simulink model "uart_xy_wiggler"  (R2018a)
settings: Solver=FixedStepDiscrete  StartTime=0.0  StopTime=inf  RelTol=1e-3
PreLoadFcn:
  | waijung.modelPreload; % Required for working with Waijung Blockset. Do not remove.
undefined symbols (not defined in the file or in its folder): HSEOSC, Link, LQFP144, ST, STM32F446ZE
libraries: simulink x10, commsynccomp2 x7, stm32f4_io_lib x3, dspstat3 x2, stm32f4_device_config_lib x1, dspbuff3 x1
(part 1 of 9)
CloseFcn:
  | waijung.modelClose; % Required for working with Waijung Blockset. Do not remove.
settings Model: Creator=Krisada  LastModifiedBy=mp
settings DataIOCC: LimitDataPoints=on  SaveFormat=Array  SignalLoggingSaveFormat=ModelDataLogs
settings OptimizationCC: ExpressionDepthLimit=2147483647  LifeSpan=1
settings DebuggingCC: UnderspecifiedInitializationDetection=Classic  MergeDetectMultiDrivingBlocksExec=none  SolverPrmCheckMsg=warning  FcnCallInpInsideContextMsg=warning  StateNameClashWarn=warning  SFUnexpectedBacktrackingDiag=warning  SFNoUnconditionalDefaultTransitionDiag=warning  SFExecutionAtInitializationDiag=none
settings HardwareCC: ProdBitPerPointer=32  ProdBitPerSizeT=32  ProdBitPerPtrDiffT=32  ProdLargestAtomicFloat=None  ProdIntDivRoundTo=Undefined  ProdWordSize=32  ProdHWDeviceType=ARM Compatible->Cortex - M4  TargetEndianess=LittleEndian  TargetHWDeviceType=ARM Compatible->Cortex - M4
settings ModelReferenceCC: PropagateSignalLabelsOutOfModel=off
settings SFSimCC: MATLABDynamicMemAlloc=off
settings RTWCC: SystemTargetFile=stm32f4.tlc  GenerateMakefile=off  TemplateMakefile=ert_default_tmf  Description=STM32F4 Target
settings CodeAppCC: IgnoreCustomStorageClasses=off  CustomSymbolStrType=$N$R$M  StateflowObjectComments=on  InternalIdentifier=Classic
settings STFCustomTargetCC: ModelReferenceCompliant=off  CombineOutputUpdateFcns=on  ERTCustomFileBanners=on  SupportContinuousTime=off  SupportNonInlinedSFcns=off  RemoveResetFunc=on  MATLABClassNameForMDSCustomization=Simulink.SoftwareTarget.ERTCustomization  GRTInterface=off  SystemTargetFile=stm32f4.tlc
settings ERTTargetCC: MultiwordLength=2048  ModelReferenceCompliant=off  ParMdlRefBuildCompliant=off  CompOptLevelCompliant=off  ConcurrentExecutionCompliant=off  ModelStepFunctionPrototypeControlCompliant=off  CPPClassGenCompliant=off  UseToolchainInfoCompliant=off  ExtModeMexFile=noextcomm  ERTSrcFileBannerTemplate=stm32f4_code_template.cgt  ERTHdrFileBannerTemplate=stm32f4_code_template.cgt  ERTDataSrcFileTemplate=stm32f4_code_template.cgt  ERTDataHdrFileTemplate=stm32f4_code_template.cgt  ERTCustomFileTemplate=stm32f4_file_process.tlc  ConvertIfToSwitch=off  SuppressUnreachableDefaultCases=off
settings ConfigComp: CovMetricSettings=dw  CovHtmlReporting=on  CovSaveCumulativeToWorkspaceVar=on  CovSaveSingleToWorkspaceVar=on  CovExternalEMLEnable=off

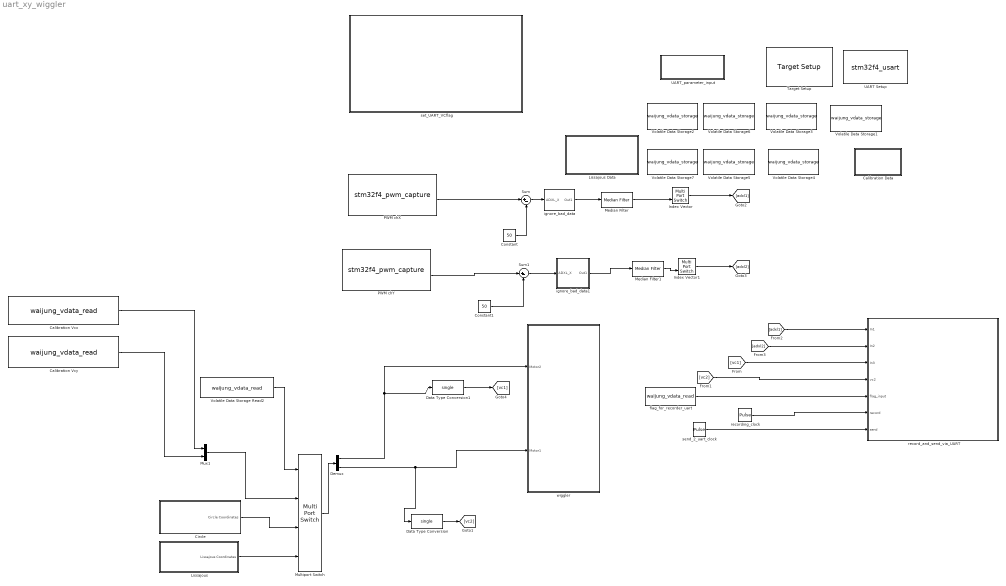
== system uart_xy_wiggler ==
  Calibration Data : Subsystem
  Calibration Vcx : S-Function  FunctionName=waijung_vdata_read  Parameters=storagename,varname,sampletime,sampletimestr,blockid,storagetype,storagetypestr  SFunctionDeploymentMode=off  EnableBusSupport=off  mask(waijung_vdata_read){storagename=vcx, varname=VolatileDataStorage2_vcx, sampletime=.01, sampletimestr=-1, blockid=CalibrationVcx, storagetype=double, storagetypestr=double}
      mask prompts: storagename "Storage Name"; varname "Variable name"; sampletime "Sample time (sec)"; sampletimestr "Compiled sample time (sec) in string"; storagetype "Data type"; storagetypestr "Data type string"
      mask help: This block implements read data from a buffer.
      mask init:
      | waijung_vdata_read_callback('init');
      mask Help: web(fullfile(waijungdocroot,'Volatile_Data_Storage_Read.htm'))
      mask TypeOptions storagename: ab3 | ab1 | ab2 | ab4 | ab5 | ab6 | ab7 | ab8 | ab9 | ab10 | Ays | Ayc | Axs | A_Laser | LissaFreq | Axc | Laser | vcx | flag | CircleFlag | CircleFrequency | vcy | CircleR
      mask Callback storagename: waijung_vdata_read_callback('storagename');
      mask Callback varname: waijung_vdata_read_callback('varname');
      mask Callback sampletime: waijung_vdata_read_callback('sampletime');
      mask Callback sampletimestr: waijung_vdata_read_callback('sampletimestr');
      mask Callback blockid: waijung_vdata_read_callback('blockid');
      mask Callback storagetype: waijung_vdata_read_callback('storagetype');
      mask Display: text(0.05, 0.5, 'Buffer: vcx','ver','middle','hor','left');port_label('output',1,'D1(double)')
  Calibration Vcy : S-Function  FunctionName=waijung_vdata_read  Parameters=storagename,varname,sampletime,sampletimestr,blockid,storagetype,storagetypestr  SFunctionDeploymentMode=off  EnableBusSupport=off  mask(waijung_vdata_read){storagename=vcy, varname=VolatileDataStorage6_vcy, sampletime=.01, sampletimestr=-1, blockid=CalibrationVcy, storagetype=double, storagetypestr=double}
      mask prompts: storagename "Storage Name"; varname "Variable name"; sampletime "Sample time (sec)"; sampletimestr "Compiled sample time (sec) in string"; storagetype "Data type"; storagetypestr "Data type string"
      mask help: This block implements read data from a buffer.
      mask init:
      | waijung_vdata_read_callback('init');
      mask Help: web(fullfile(waijungdocroot,'Volatile_Data_Storage_Read.htm'))
      mask TypeOptions storagename: ab3 | ab1 | ab2 | ab4 | ab5 | ab6 | ab7 | ab8 | ab9 | ab10 | Ays | Ayc | Axs | A_Laser | LissaFreq | Axc | Laser | vcx | flag | CircleFlag | CircleFrequency | vcy | CircleR
      mask Callback storagename: waijung_vdata_read_callback('storagename');
      mask Callback varname: waijung_vdata_read_callback('varname');
      mask Callback sampletime: waijung_vdata_read_callback('sampletime');
      mask Callback sampletimestr: waijung_vdata_read_callback('sampletimestr');
      mask Callback blockid: waijung_vdata_read_callback('blockid');
      mask Callback storagetype: waijung_vdata_read_callback('storagetype');
      mask Display: text(0.05, 0.5, 'Buffer: vcy','ver','middle','hor','left');port_label('output',1,'D1(double)')
  Circle : Subsystem
  Constant : Constant  Value=50  OutDataTypeStr=single
  Constant1 : Constant  Value=50  OutDataTypeStr=single
  Data Type Conversion : DataTypeConversion  OutDataTypeStr=single
  Data Type Conversion1 : DataTypeConversion  OutDataTypeStr=single
  Demux : Demux  Outputs=2
  Index Vector : MultiPortSwitch  DataPortOrder=Zero-based contiguous  Inputs=1  zeroidx=on
  Index Vector1 : MultiPortSwitch  DataPortOrder=Zero-based contiguous  Inputs=1  zeroidx=on
  Lissajous : Subsystem
  Lissajous Data : Subsystem
  Median Filter : dspstat3/Median Filter  WindowLength=5  SimulateUsing=Interpreted execution
      settings: SourceProductName=DSP System Toolbox  SourceProductBaseCode=DS
  Median Filter1 : dspstat3/Median Filter  WindowLength=5  SimulateUsing=Interpreted execution
      settings: SourceProductName=DSP System Toolbox  SourceProductBaseCode=DS
  Multiport Switch : MultiPortSwitch  DataPortOrder=Zero-based contiguous  zeroidx=on
  Mux1 : Mux  Inputs=2
  PWM chX : S-Function  FunctionName=stm32f4_pwm_capture  Parameters=conf,inputporttype,inputportwidth,outputporttype,outputportwidth,optionstring,sampletime,blockid  SFunctionDeploymentMode=off  EnableBusSupport=off  mask(stm32f4_pwm_capture){conf=Capture, timer=2, lasttimer=2, pin=B3, pintype=Pull Up, edge=Rising, datatype=single, portpinstr=0, sampletime=0.01, blockid=PWMchX, inputporttype=[], inputportwidth=[], inputportlabel={}, outputporttype=[3 1 1 1], outputportwidth=[], outputportlabel={'READY','+Width (sec)','+Duty (%)','Frequency (Hz)'}, compat=0, optionstring=["2","1","B","3","2","32","Rising","UP","float"]}
      mask prompts: conf "Configuration"; lasttimer "Last Timer"; pin "Capture Pin"; pintype "Capture Pin Type (Pull-Up/Pull-Down)"; edge "Capture Edge"; datatype "Output data type"; portpinstr "Port Pin String"; sampletime "Sample time (sec)"; blockid "Block ID"; inputporttype "Input Port Type"; inputportwidth "Input Port Width"; inputportlabel "Input Port Label"; outputporttype "Output Port Type"; outputportwidth "Output Port Width"; outputportlabel "Output port label"; compat "Compatibility (Reserved for future use)"; optionstring "String(s) to be passed to TLC"
      mask help:
      | Capture Edge:
      |  Rising - PWM period start from rising edge of pulse N to rising edge of pulse N+1
      |  Falling - PWM period start from falling edge of pulse N to falling edge of pulse N+1
      | Capture data type:
      |  Capture data type, selectable to double or single.
      |
      | Output:
      |  READY - indicate the status of capture, a non-zero value indicate data is ready.
      |  +Width - positive pulse width, in unit of second.
      |  +Duty - positive duty cycle, 0 to 100%
      |  Frequency - signal frequency in unit of Hz
      |
      | Note: caprure period should not longer than 1 second (Maximum limit is 3 seconds)
      mask init:
      | stm32f4_pwm_capture_callback('init');
      mask Help: web(fullfile(waijungdocroot,'stm32f4_pwm_capture.htm'), '-browser')
      mask TypeOptions conf: Capture
      mask Callback conf: stm32f4_pwm_capture_callback('conf');
      mask TypeOptions timer: 1 | 2 | 3 | 4 | 5 | 8
      mask Callback timer: stm32f4_pwm_capture_callback('timer');
      mask TypeOptions pin: Not used | A0 | A5 | A15 | A1 | B3 | A2 | B10 | A3 | B11
      mask TypeOptions pintype: None | Pull Up | Pull Down
      mask TypeOptions edge: Rising | Falling
      mask TypeOptions datatype: double | single
      mask Callback sampletime: stm32f4_pwm_capture_callback('sampletime');
      mask Callback blockid: stm32f4_pwm_capture_callback('blockid');
      mask Display: text(0.05, 0.5, 'Timer: 2 (32 bit)\nInput Pin: B3\nEdge: Rising\nTs (sec): -1','ver','middle','hor','left'); port_label('output', 1,'READY'); port_label('output', 2,'+Width (sec)'); port_label('output', 3,'+Duty (%)'); port_label('output', 4,'Frequency (Hz)');
  PWM chY : S-Function  FunctionName=stm32f4_pwm_capture  Parameters=conf,inputporttype,inputportwidth,outputporttype,outputportwidth,optionstring,sampletime,blockid  SFunctionDeploymentMode=off  EnableBusSupport=off  mask(stm32f4_pwm_capture){conf=Capture, timer=5, lasttimer=5, pin=A0, pintype=Pull Up, edge=Rising, datatype=single, portpinstr=0, sampletime=0.01, blockid=PWMchY, inputporttype=[], inputportwidth=[], inputportlabel={}, outputporttype=[3 1 1 1], outputportwidth=[], outputportlabel={'READY','+Width (sec)','+Duty (%)','Frequency (Hz)'}, compat=0, optionstring=["5","1","A","0","1","32","Rising","UP","float"]}
      mask prompts: conf "Configuration"; lasttimer "Last Timer"; pin "Capture Pin"; pintype "Capture Pin Type (Pull-Up/Pull-Down)"; edge "Capture Edge"; datatype "Output data type"; portpinstr "Port Pin String"; sampletime "Sample time (sec)"; blockid "Block ID"; inputporttype "Input Port Type"; inputportwidth "Input Port Width"; inputportlabel "Input Port Label"; outputporttype "Output Port Type"; outputportwidth "Output Port Width"; outputportlabel "Output port label"; compat "Compatibility (Reserved for future use)"; optionstring "String(s) to be passed to TLC"
      mask help:
      | Capture Edge:
      |  Rising - PWM period start from rising edge of pulse N to rising edge of pulse N+1
      |  Falling - PWM period start from falling edge of pulse N to falling edge of pulse N+1
      | Capture data type:
      |  Capture data type, selectable to double or single.
      |
      | Output:
      |  READY - indicate the status of capture, a non-zero value indicate data is ready.
      |  +Width - positive pulse width, in unit of second.
      |  +Duty - positive duty cycle, 0 to 100%
      |  Frequency - signal frequency in unit of Hz
      |
      | Note: caprure period should not longer than 1 second (Maximum limit is 3 seconds)
      mask init:
      | stm32f4_pwm_capture_callback('init');
      mask Help: web(fullfile(waijungdocroot,'stm32f4_pwm_capture.htm'), '-browser')
      mask TypeOptions conf: Capture
      mask Callback conf: stm32f4_pwm_capture_callback('conf');
      mask TypeOptions timer: 1 | 2 | 3 | 4 | 5 | 8
      mask Callback timer: stm32f4_pwm_capture_callback('timer');
      mask TypeOptions pin: Not used | A0 | A1 | A2 | A3
      mask TypeOptions pintype: None | Pull Up | Pull Down
      mask TypeOptions edge: Rising | Falling
      mask TypeOptions datatype: double | single
      mask Callback sampletime: stm32f4_pwm_capture_callback('sampletime');
      mask Callback blockid: stm32f4_pwm_capture_callback('blockid');
      mask Display: text(0.05, 0.5, 'Timer: 5 (32 bit)\nInput Pin: A0\nEdge: Rising\nTs (sec): -1','ver','middle','hor','left'); port_label('output', 1,'READY'); port_label('output', 2,'+Width (sec)'); port_label('output', 3,'+Duty (%)'); port_label('output', 4,'Frequency (Hz)');
  Sum : Sum  Inputs=|+-
  Sum1 : Sum  Inputs=|+-
  Target Setup : stm32f4_device_config_lib/Target Setup  Priority=1  compiler=GNU ARM  previous_compiler=GNU ARM  mcu=STM32F446ZE (LQFP144)  mcustr=STM32F446ZE  clockconfig=HSEOSC-8MHz  system_stm32f4xx_c_path=C:\MATLAB\waijung17_03a\targets\stm32f4_target\stm32f4\utils\system_stm32f4xx_default\STM32F446xx\hseosc8mhz  showmemoryconfiguration=off  stacksize=0x400  heapsize=0x200  enableautocompiledownload=on  fullchiperase=off  programmerinterface=ST-Link  editctrlstr=on  compilercontrolstr=$(patsubst %, -I%, .) -mcpu=cortex-m4 -mthumb -mthumb-interwork -mfloat-abi=hard -mfpu=fpv4-sp-d16 -ffast-math -Wall -Wextra -Ofast  assemblercontrolstr=$(patsubst %, -I%, .) -mcpu=cortex-m4 -mthumb -mthumb-interwork -mfloat-abi=hard -mfpu=fpv4-sp-d16 -ffast-math -Wall -Wextra -Ofast -Wa,-amhls=$(<:.s=.lst) -D__STACK_SIZE=$(STACK_SIZE) -D__HEAP_SIZE=$(HEAP_SIZE)  linkercontrolstr=-T$(LD_SCRIPT) -g -Wl,-Map=$(MAP),--cref,--no-warn-mismatch -mcpu=cortex-m4 -mthumb -mthumb-interwork -mfloat-abi=hard -mfpu=fpv4-sp-d16 -specs=nosys.specs  runafterdownload=on  execprofile=None  profileruart=1  profilerbaud=115200  profilertxpin=D8  profilerinitstr=0.001,180000000,180000,115200,0  manualsetsampletime=on  sampletime=0.001  blockid=TargetSetup  systickreloadvalue=180000  hseval=8000000  lastprofileruart=1  hclk=180000000  flashorigin=0x8000000  flashlength=512k  ramorigin=0x20000000  ramlength=128k  useextram=off
      settings: SourceProductName=Waijung Blockset
  UART Setup : S-Function  Priority=1  FunctionName=stm32f4_usart  Parameters=configuration,uartmodule,transfer,baudrate,inputtype,outputtype,confstr,binheaderarray,binterminatorarray,asciiheader,asciiterminator,bindatalength,packetmode,varname,sampletime,sampletimestr,blockid  SFunctionDeploymentMode=off  EnableBusSupport=off  mask(stm32f4_usart){configuration=Setup, uartmodule=3, baudrate=115200, databits=8, parity=No, stopbit=1, remaptxpin=D8, remaprxpin=D9, flowcontrol=None, remapctspin=Not used, remaprtspin=Not used, advanceoptions=off, rxbuffersize=512, txbuffersize=512, transfer=Blocking, packetmode=Ascii, binheader='7E 7E', binterminator='03 03', porttype_double=1, porttype_single=0, porttype_int8=1, porttype_uint8=0, porttype_int16=0, porttype_uint16=0, porttype_int32=0, porttype_uint32=0, asciiformat='%d,%f', rx_asciiterminator=CRLF (0x0D 0x0A - "\r\n"), tx_asciiterminator=CR (0x0D - "\r"), storagename=<empty>, varname=, inputtype=[0], outputtype=[0], binheaderarray=[0], binterminatorarray=[0], bindatalength=0, asciiheader='', asciiterminator=[0], sampletime=-1, sampletimestr=-1, blockid=UARTSetup, confstr=[ "dummy", "1", "D", "8", "1", "D", "9", "0", "*", "*", "0", "*", "*", "1", "4", "3", "1", "4", "1", "512", "512", "1", "3", "115200", "8", "No", "1", "None", "USART3"], lastmodule=3}
      mask prompts: uartmodule "UART Module"; baudrate "Baud rate (bps)"; databits "Data bits"; stopbit "Stop bit"; remaptxpin "Tx Pin"; remaprxpin "Rx Pin"; flowcontrol "Hardware flow control"; remapctspin "HW Flow control, CTS Pin"; remaprtspin "HW Flow control, RTS Pin"; advanceoptions "Advance options"; rxbuffersize "Rx buffer size (bytes)"; txbuffersize "Tx buffer size (bytes)"; packetmode "Packet mode"; binheader "Binary header (example: '7E 7E')"; binterminator "Binary terminator (example: '03 03')"; porttype_double "Number of data port, type DOUBLE"; porttype_single "Number of data port, type SINGLE"; porttype_int8 "Number of data port, type INT8"; porttype_uint8 "Number of data port, type UINT8"; porttype_int16 "Number of data port, type INT16"; porttype_uint16 "Number of data port, type UINT16"; porttype_int32 "Number of data port, type INT32"; porttype_uint32 "Number of data port, type UINT32"; asciiformat "Ascii format"; rx_asciiterminator "End of packet"; tx_asciiterminator "End of packet"; storagename "Buffer"; varname "Var name"; inputtype "Input data type"; outputtype "Output data type"; binheaderarray "Binary header"; binterminatorarray "Binary terminator"; bindatalength "Binary data length"; asciiheader "Ascii header (printf format)"; asciiterminator "Ascii terminator"; sampletime "Sample time (sec)"; sampletimestr "Compiled sample time (sec) in string"; confstr "Configuration string"; lastmodule "Last module selected"
      mask init:
      | stm32f4_usart_callback('init');
      mask Help: web(fullfile(waijungdocroot,'stm32f4_usart_setup.htm'), '-browser')
      mask TypeOptions configuration: Setup | Tx | Rx
      mask Callback configuration: stm32f4_usart_callback('configuration');
      mask TypeOptions uartmodule: 1 | 2 | 3 | 4 | 5 | 6
      mask Callback uartmodule: stm32f4_usart_callback('uartmodule');
      mask Callback baudrate: stm32f4_usart_callback('baudrate');
      mask TypeOptions databits: 8
      mask TypeOptions parity: No | Odd | Even
      mask TypeOptions stopbit: 0.5 | 1 | 1.5 | 2
      mask TypeOptions remaptxpin: Not used | B10 | C10 | D8
      mask TypeOptions remaprxpin: Not used | B11 | C11 | D9
      mask TypeOptions flowcontrol: None | RTS | CTS | RTS/CTS
      mask Callback flowcontrol: stm32f4_usart_callback('flowcontrol');
      mask TypeOptions remapctspin: Not used | B13 | D11
      mask TypeOptions remaprtspin: Not used | B14 | D12
      mask Callback advanceoptions: stm32f4_usart_callback('advanceoptions');
      mask TypeOptions rxbuffersize: 16 | 32 | 64 | 128 | 256 | 512 | 1024 | 2048
      mask TypeOptions txbuffersize: 16 | 32 | 64 | 128 | 256 | 512 | 1024 | 2048
      mask TypeOptions transfer: Blocking | Non-Blocking
      mask Callback transfer: stm32f4_usart_callback('transfer');
      mask TypeOptions packetmode: Ascii | Binary | String Buffer
      mask Callback packetmode: stm32f4_usart_callback('packetmode');
      mask Callback binheader: stm32f4_usart_callback('binheader');
      mask Callback binterminator: stm32f4_usart_callback('binterminator');
      mask Callback porttype_double: stm32f4_usart_callback('porttype');
      mask Callback porttype_single: stm32f4_usart_callback('porttype');
      mask Callback porttype_int8: stm32f4_usart_callback('porttype');
      mask Callback porttype_uint8: stm32f4_usart_callback('porttype');
      mask Callback porttype_int16: stm32f4_usart_callback('porttype');
      mask Callback porttype_uint16: stm32f4_usart_callback('porttype');
      mask Callback porttype_int32: stm32f4_usart_callback('porttype');
      mask Callback porttype_uint32: stm32f4_usart_callback('porttype');
      mask Callback asciiformat: stm32f4_usart_callback('asciiformat');
      mask TypeOptions rx_asciiterminator: CR (0x0D - "\r") | LF (0x0A - "\n") | CRLF (0x0D 0x0A - "\r\n")
      mask Callback rx_asciiterminator: stm32f4_usart_callback('rx_asciiterminator');
      mask TypeOptions tx_asciiterminator: CR (0x0D - "\r") | LF (0x0A - "\n") | CRLF (0x0D 0x0A - "\r\n") | None
      mask Callback tx_asciiterminator: stm32f4_usart_callback('tx_asciiterminator');
      mask TypeOptions storagename: <empty>
      mask Callback storagename: stm32f4_usart_callback('storagename');
      mask Callback varname: stm32f4_usart_callback('varname');
      mask Callback sampletime: stm32f4_usart_callback('sampletime');
      mask Callback sampletimestr: stm32f4_usart_callback('sampletimestr');
      mask Callback blockid: stm32f4_usart_callback('blockid');
      mask Display: text(0.5, 0.5, 'Module: USART3_Setup\nBaud (Bps): 115200\nDMA Buffer: 512/512\nTx/Rx Pin: D8/D9','ver','middle','hor','center');
  UART_parameter_input : Subsystem
  Volatile Data Storage Read2 : S-Function  FunctionName=waijung_vdata_read  Parameters=storagename,varname,sampletime,sampletimestr,blockid,storagetype,storagetypestr  SFunctionDeploymentMode=off  EnableBusSupport=off  mask(waijung_vdata_read){storagename=CircleFlag, varname=VolatileDataStorage4_CircleFlag, sampletime=.01, sampletimestr=-1, blockid=VolatileDataStorageRead2, storagetype=double, storagetypestr=double}
      mask prompts: storagename "Storage Name"; varname "Variable name"; sampletime "Sample time (sec)"; sampletimestr "Compiled sample time (sec) in string"; storagetype "Data type"; storagetypestr "Data type string"
      mask help: This block implements read data from a buffer.
      mask init:
      | waijung_vdata_read_callback('init');
      mask Help: web(fullfile(waijungdocroot,'Volatile_Data_Storage_Read.htm'))
      mask TypeOptions storagename: ab3 | ab1 | ab2 | ab4 | ab5 | ab6 | ab7 | ab8 | ab9 | ab10 | Ays | Ayc | Axs | A_Laser | LissaFreq | Axc | Laser | vcx | flag | CircleFlag | CircleFrequency | vcy | CircleR
      mask Callback storagename: waijung_vdata_read_callback('storagename');
      mask Callback varname: waijung_vdata_read_callback('varname');
      mask Callback sampletime: waijung_vdata_read_callback('sampletime');
      mask Callback sampletimestr: waijung_vdata_read_callback('sampletimestr');
      mask Callback blockid: waijung_vdata_read_callback('blockid');
      mask Callback storagetype: waijung_vdata_read_callback('storagetype');
      mask Display: text(0.05, 0.5, 'Buffer: CircleFlag','ver','middle','hor','left');port_label('output',1,'D1(double)')
  Volatile Data Storage1 : S-Function  FunctionName=waijung_vdata_storage  Parameters=storagetype,storagename,initval,varname,buffersize,initvalstring,sampletime,sampletimestr,blockid,storagetypestr  SFunctionDeploymentMode=off  EnableBusSupport=off  mask(waijung_vdata_storage){storagetype=single, definevolatile=on, storagename=Laser, initval=90, varname=VolatileDataStorage1_Laser, buffersize=64, initvalstring='Initial string', webintegration=Disable, weboutputformat='%f', webcgicallback=(void*)0, laststoragetype=single, sampletime=-1, sampletimestr=-1, blockid=VolatileDataStorage1, storagetypestr=volatile float}
      mask prompts: storagetype "Storage Type"; definevolatile "Define with "volatile" keyword"; storagename "Storage Name (must be a valid variable name)"; initval "Initial value (Apply at Power on Reset only)"; varname "Variable name"; buffersize "Size (bytes)"; initvalstring "Initial value (Apply at Power on Reset only)"; webintegration "Web CGI varget/varset integration"; weboutputformat "Web CGI varget output format"; webcgicallback "Web CGI varset callback"; laststoragetype "Last selected Storage Type"; sampletime "Sample time (sec)"; sampletimestr "Compiled sample time (sec) in string"; storagetypestr "Type string"
      mask help:
      | This block implements a volatile Data Storage.
      |
      | Web CGI varset/varget integratiopn:
      | Enable - In webserver application, allow remote access via http.
      | Disable - Variable is use in local only.
      mask init:
      | waijung_vdata_storage_callback('init');
      mask Help: web(fullfile(waijungdocroot,'Volatile_Data_Storage.htm'))
      mask TypeOptions storagetype: double | single | uint32 | int32 | uint16 | int16 | uint8 | int8 | string
      mask Callback storagetype: waijung_vdata_storage_callback('storagetype');
      mask Callback storagename: waijung_vdata_storage_callback('storagename');
      mask Callback initval: waijung_vdata_storage_callback('initval');
      mask Callback varname: waijung_vdata_storage_callback('varname');
      mask Callback initvalstring: waijung_vdata_storage_callback('initvalstring');
      mask TypeOptions webintegration: Disable | ReadOnly | Write/ Read | ReadOnly with KeyValuePair | Write/ Read with KeyValuePair
      mask Callback webintegration: waijung_vdata_storage_callback('webintegration');
      mask Callback weboutputformat: waijung_vdata_storage_callback('weboutputformat');
      mask TypeOptions laststoragetype: double | single | uint32 | int32 | uint16 | int16 | uint8 | int8 | string
      mask Callback sampletime: waijung_vdata_storage_callback('sampletime');
      mask Callback sampletimestr: waijung_vdata_storage_callback('sampletimestr');
      mask Callback blockid: waijung_vdata_storage_callback('blockid');
      mask Display: text(0.5, 0.5, 'Name: Laser\nType: single','ver','middle','hor','center')
  Volatile Data Storage2 : S-Function  FunctionName=waijung_vdata_storage  Parameters=storagetype,storagename,initval,varname,buffersize,initvalstring,sampletime,sampletimestr,blockid,storagetypestr  SFunctionDeploymentMode=off  EnableBusSupport=off  mask(waijung_vdata_storage){storagetype=double, definevolatile=on, storagename=vcx, initval=0, varname=VolatileDataStorage2_vcx, buffersize=64, initvalstring='Initial string', webintegration=Disable, weboutputformat='%f', webcgicallback=(void*)0, laststoragetype=double, sampletime=-1, sampletimestr=-1, blockid=VolatileDataStorage2, storagetypestr=volatile double}
      mask prompts: storagetype "Storage Type"; definevolatile "Define with "volatile" keyword"; storagename "Storage Name (must be a valid variable name)"; initval "Initial value (Apply at Power on Reset only)"; varname "Variable name"; buffersize "Size (bytes)"; initvalstring "Initial value (Apply at Power on Reset only)"; webintegration "Web CGI varget/varset integration"; weboutputformat "Web CGI varget output format"; webcgicallback "Web CGI varset callback"; laststoragetype "Last selected Storage Type"; sampletime "Sample time (sec)"; sampletimestr "Compiled sample time (sec) in string"; storagetypestr "Type string"
      mask help:
      | This block implements a volatile Data Storage.
      |
      | Web CGI varset/varget integratiopn:
      | Enable - In webserver application, allow remote access via http.
      | Disable - Variable is use in local only.
      mask init:
      | waijung_vdata_storage_callback('init');
      mask Help: web(fullfile(waijungdocroot,'Volatile_Data_Storage.htm'))
      mask TypeOptions storagetype: double | single | uint32 | int32 | uint16 | int16 | uint8 | int8 | string
      mask Callback storagetype: waijung_vdata_storage_callback('storagetype');
      mask Callback storagename: waijung_vdata_storage_callback('storagename');
      mask Callback initval: waijung_vdata_storage_callback('initval');
      mask Callback varname: waijung_vdata_storage_callback('varname');
      mask Callback initvalstring: waijung_vdata_storage_callback('initvalstring');
      mask TypeOptions webintegration: Disable | ReadOnly | Write/ Read | ReadOnly with KeyValuePair | Write/ Read with KeyValuePair
      mask Callback webintegration: waijung_vdata_storage_callback('webintegration');
      mask Callback weboutputformat: waijung_vdata_storage_callback('weboutputformat');
      mask TypeOptions laststoragetype: double | single | uint32 | int32 | uint16 | int16 | uint8 | int8 | string
      mask Callback sampletime: waijung_vdata_storage_callback('sampletime');
      mask Callback sampletimestr: waijung_vdata_storage_callback('sampletimestr');
      mask Callback blockid: waijung_vdata_storage_callback('blockid');
      mask Display: text(0.5, 0.5, 'Name: vcx\nType: double','ver','middle','hor','center')
  Volatile Data Storage3 : S-Function  FunctionName=waijung_vdata_storage  Parameters=storagetype,storagename,initval,varname,buffersize,initvalstring,sampletime,sampletimestr,blockid,storagetypestr  SFunctionDeploymentMode=off  EnableBusSupport=off  mask(waijung_vdata_storage){storagetype=uint8, definevolatile=on, storagename=flag, initval=0, varname=VolatileDataStorage3_flag, buffersize=64, initvalstring='Initial string', webintegration=Disable, weboutputformat='%u', webcgicallback=(void*)0, laststoragetype=uint8, sampletime=-1, sampletimestr=-1, blockid=VolatileDataStorage3, storagetypestr=volatile uint8_t}
      mask prompts: storagetype "Storage Type"; definevolatile "Define with "volatile" keyword"; storagename "Storage Name (must be a valid variable name)"; initval "Initial value (Apply at Power on Reset only)"; varname "Variable name"; buffersize "Size (bytes)"; initvalstring "Initial value (Apply at Power on Reset only)"; webintegration "Web CGI varget/varset integration"; weboutputformat "Web CGI varget output format"; webcgicallback "Web CGI varset callback"; laststoragetype "Last selected Storage Type"; sampletime "Sample time (sec)"; sampletimestr "Compiled sample time (sec) in string"; storagetypestr "Type string"
      mask help:
      | This block implements a volatile Data Storage.
      |
      | Web CGI varset/varget integratiopn:
      | Enable - In webserver application, allow remote access via http.
      | Disable - Variable is use in local only.
      mask init:
      | waijung_vdata_storage_callback('init');
      mask Help: web(fullfile(waijungdocroot,'Volatile_Data_Storage.htm'))
      mask TypeOptions storagetype: double | single | uint32 | int32 | uint16 | int16 | uint8 | int8 | string
      mask Callback storagetype: waijung_vdata_storage_callback('storagetype');
      mask Callback storagename: waijung_vdata_storage_callback('storagename');
      mask Callback initval: waijung_vdata_storage_callback('initval');
      mask Callback varname: waijung_vdata_storage_callback('varname');
      mask Callback initvalstring: waijung_vdata_storage_callback('initvalstring');
      mask TypeOptions webintegration: Disable | ReadOnly | Write/ Read | ReadOnly with KeyValuePair | Write/ Read with KeyValuePair
      mask Callback webintegration: waijung_vdata_storage_callback('webintegration');
      mask Callback weboutputformat: waijung_vdata_storage_callback('weboutputformat');
      mask TypeOptions laststoragetype: double | single | uint32 | int32 | uint16 | int16 | uint8 | int8 | string
      mask Callback sampletime: waijung_vdata_storage_callback('sampletime');
      mask Callback sampletimestr: waijung_vdata_storage_callback('sampletimestr');
      mask Callback blockid: waijung_vdata_storage_callback('blockid');
      mask Display: text(0.5, 0.5, 'Name: flag\nType: uint8','ver','middle','hor','center')
  Volatile Data Storage4 : S-Function  FunctionName=waijung_vdata_storage  Parameters=storagetype,storagename,initval,varname,buffersize,initvalstring,sampletime,sampletimestr,blockid,storagetypestr  SFunctionDeploymentMode=off  EnableBusSupport=off  mask(waijung_vdata_storage){storagetype=double, definevolatile=on, storagename=CircleFlag, initval=0, varname=VolatileDataStorage4_CircleFlag, buffersize=64, initvalstring='Initial string', webintegration=Disable, weboutputformat='%f', webcgicallback=(void*)0, laststoragetype=double, sampletime=-1, sampletimestr=-1, blockid=VolatileDataStorage4, storagetypestr=volatile double}
      mask prompts: storagetype "Storage Type"; definevolatile "Define with "volatile" keyword"; storagename "Storage Name (must be a valid variable name)"; initval "Initial value (Apply at Power on Reset only)"; varname "Variable name"; buffersize "Size (bytes)"; initvalstring "Initial value (Apply at Power on Reset only)"; webintegration "Web CGI varget/varset integration"; weboutputformat "Web CGI varget output format"; webcgicallback "Web CGI varset callback"; laststoragetype "Last selected Storage Type"; sampletime "Sample time (sec)"; sampletimestr "Compiled sample time (sec) in string"; storagetypestr "Type string"
      mask help:
      | This block implements a volatile Data Storage.
      |
      | Web CGI varset/varget integratiopn:
      | Enable - In webserver application, allow remote access via http.
      | Disable - Variable is use in local only.
      mask init:
      | waijung_vdata_storage_callback('init');
      mask Help: web(fullfile(waijungdocroot,'Volatile_Data_Storage.htm'))
      mask TypeOptions storagetype: double | single | uint32 | int32 | uint16 | int16 | uint8 | int8 | string
      mask Callback storagetype: waijung_vdata_storage_callback('storagetype');
      mask Callback storagename: waijung_vdata_storage_callback('storagename');
      mask Callback initval: waijung_vdata_storage_callback('initval');
      mask Callback varname: waijung_vdata_storage_callback('varname');
      mask Callback initvalstring: waijung_vdata_storage_callback('initvalstring');
      mask TypeOptions webintegration: Disable | ReadOnly | Write/ Read | ReadOnly with KeyValuePair | Write/ Read with KeyValuePair
      mask Callback webintegration: waijung_vdata_storage_callback('webintegration');
      mask Callback weboutputformat: waijung_vdata_storage_callback('weboutputformat');
      mask TypeOptions laststoragetype: double | single | uint32 | int32 | uint16 | int16 | uint8 | int8 | string
      mask Callback sampletime: waijung_vdata_storage_callback('sampletime');
      mask Callback sampletimestr: waijung_vdata_storage_callback('sampletimestr');
      mask Callback blockid: waijung_vdata_storage_callback('blockid');
      mask Display: text(0.5, 0.5, 'Name: CircleFlag\nType: double','ver','middle','hor','center')
  Volatile Data Storage5 : S-Function  FunctionName=waijung_vdata_storage  Parameters=storagetype,storagename,initval,varname,buffersize,initvalstring,sampletime,sampletimestr,blockid,storagetypestr  SFunctionDeploymentMode=off  EnableBusSupport=off  mask(waijung_vdata_storage){storagetype=double, definevolatile=on, storagename=CircleFrequency, initval=0.1, varname=VolatileDataStorage5_CircleFrequency, buffersize=64, initvalstring='Initial string', webintegration=Disable, weboutputformat='%f', webcgicallback=(void*)0, laststoragetype=double, sampletime=-1, sampletimestr=-1, blockid=VolatileDataStorage5, storagetypestr=volatile double}
      mask prompts: storagetype "Storage Type"; definevolatile "Define with "volatile" keyword"; storagename "Storage Name (must be a valid variable name)"; initval "Initial value (Apply at Power on Reset only)"; varname "Variable name"; buffersize "Size (bytes)"; initvalstring "Initial value (Apply at Power on Reset only)"; webintegration "Web CGI varget/varset integration"; weboutputformat "Web CGI varget output format"; webcgicallback "Web CGI varset callback"; laststoragetype "Last selected Storage Type"; sampletime "Sample time (sec)"; sampletimestr "Compiled sample time (sec) in string"; storagetypestr "Type string"
      mask help:
      | This block implements a volatile Data Storage.
      |
      | Web CGI varset/varget integratiopn:
      | Enable - In webserver application, allow remote access via http.
      | Disable - Variable is use in local only.
      mask init:
      | waijung_vdata_storage_callback('init');
      mask Help: web(fullfile(waijungdocroot,'Volatile_Data_Storage.htm'))
      mask TypeOptions storagetype: double | single | uint32 | int32 | uint16 | int16 | uint8 | int8 | string
      mask Callback storagetype: waijung_vdata_storage_callback('storagetype');
      mask Callback storagename: waijung_vdata_storage_callback('storagename');
      mask Callback initval: waijung_vdata_storage_callback('initval');
      mask Callback varname: waijung_vdata_storage_callback('varname');
      mask Callback initvalstring: waijung_vdata_storage_callback('initvalstring');
      mask TypeOptions webintegration: Disable | ReadOnly | Write/ Read | ReadOnly with KeyValuePair | Write/ Read with KeyValuePair
      mask Callback webintegration: waijung_vdata_storage_callback('webintegration');
      mask Callback weboutputformat: waijung_vdata_storage_callback('weboutputformat');
      mask TypeOptions laststoragetype: double | single | uint32 | int32 | uint16 | int16 | uint8 | int8 | string
      mask Callback sampletime: waijung_vdata_storage_callback('sampletime');
      mask Callback sampletimestr: waijung_vdata_storage_callback('sampletimestr');
      mask Callback blockid: waijung_vdata_storage_callback('blockid');
      mask Display: text(0.5, 0.5, 'Name: CircleFrequency\nType: double','ver','middle','hor','center')
  Volatile Data Storage6 : S-Function  FunctionName=waijung_vdata_storage  Parameters=storagetype,storagename,initval,varname,buffersize,initvalstring,sampletime,sampletimestr,blockid,storagetypestr  SFunctionDeploymentMode=off  EnableBusSupport=off  mask(waijung_vdata_storage){storagetype=double, definevolatile=on, storagename=vcy, initval=0, varname=VolatileDataStorage6_vcy, buffersize=64, initvalstring='Initial string', webintegration=Disable, weboutputformat='%f', webcgicallback=(void*)0, laststoragetype=double, sampletime=-1, sampletimestr=-1, blockid=VolatileDataStorage6, storagetypestr=volatile double}
      mask prompts: storagetype "Storage Type"; definevolatile "Define with "volatile" keyword"; storagename "Storage Name (must be a valid variable name)"; initval "Initial value (Apply at Power on Reset only)"; varname "Variable name"; buffersize "Size (bytes)"; initvalstring "Initial value (Apply at Power on Reset only)"; webintegration "Web CGI varget/varset integration"; weboutputformat "Web CGI varget output format"; webcgicallback "Web CGI varset callback"; laststoragetype "Last selected Storage Type"; sampletime "Sample time (sec)"; sampletimestr "Compiled sample time (sec) in string"; storagetypestr "Type string"
      mask help:
      | This block implements a volatile Data Storage.
      |
      | Web CGI varset/varget integratiopn:
      | Enable - In webserver application, allow remote access via http.
      | Disable - Variable is use in local only.
      mask init:
      | waijung_vdata_storage_callback('init');
      mask Help: web(fullfile(waijungdocroot,'Volatile_Data_Storage.htm'))
      mask TypeOptions storagetype: double | single | uint32 | int32 | uint16 | int16 | uint8 | int8 | string
      mask Callback storagetype: waijung_vdata_storage_callback('storagetype');
      mask Callback storagename: waijung_vdata_storage_callback('storagename');
      mask Callback initval: waijung_vdata_storage_callback('initval');
      mask Callback varname: waijung_vdata_storage_callback('varname');
      mask Callback initvalstring: waijung_vdata_storage_callback('initvalstring');
      mask TypeOptions webintegration: Disable | ReadOnly | Write/ Read | ReadOnly with KeyValuePair | Write/ Read with KeyValuePair
      mask Callback webintegration: waijung_vdata_storage_callback('webintegration');
      mask Callback weboutputformat: waijung_vdata_storage_callback('weboutputformat');
      mask TypeOptions laststoragetype: double | single | uint32 | int32 | uint16 | int16 | uint8 | int8 | string
      mask Callback sampletime: waijung_vdata_storage_callback('sampletime');
      mask Callback sampletimestr: waijung_vdata_storage_callback('sampletimestr');
      mask Callback blockid: waijung_vdata_storage_callback('blockid');
      mask Display: text(0.5, 0.5, 'Name: vcy\nType: double','ver','middle','hor','center')
  Volatile Data Storage7 : S-Function  FunctionName=waijung_vdata_storage  Parameters=storagetype,storagename,initval,varname,buffersize,initvalstring,sampletime,sampletimestr,blockid,storagetypestr  SFunctionDeploymentMode=off  EnableBusSupport=off  mask(waijung_vdata_storage){storagetype=double, definevolatile=on, storagename=CircleR, initval=0.1, varname=VolatileDataStorage7_CircleR, buffersize=64, initvalstring='Initial string', webintegration=Disable, weboutputformat='%f', webcgicallback=(void*)0, laststoragetype=double, sampletime=-1, sampletimestr=-1, blockid=VolatileDataStorage7, storagetypestr=volatile double}
      mask prompts: storagetype "Storage Type"; definevolatile "Define with "volatile" keyword"; storagename "Storage Name (must be a valid variable name)"; initval "Initial value (Apply at Power on Reset only)"; varname "Variable name"; buffersize "Size (bytes)"; initvalstring "Initial value (Apply at Power on Reset only)"; webintegration "Web CGI varget/varset integration"; weboutputformat "Web CGI varget output format"; webcgicallback "Web CGI varset callback"; laststoragetype "Last selected Storage Type"; sampletime "Sample time (sec)"; sampletimestr "Compiled sample time (sec) in string"; storagetypestr "Type string"
      mask help:
      | This block implements a volatile Data Storage.
      |
      | Web CGI varset/varget integratiopn:
      | Enable - In webserver application, allow remote access via http.
      | Disable - Variable is use in local only.
      mask init:
      | waijung_vdata_storage_callback('init');
      mask Help: web(fullfile(waijungdocroot,'Volatile_Data_Storage.htm'))
      mask TypeOptions storagetype: double | single | uint32 | int32 | uint16 | int16 | uint8 | int8 | string
      mask Callback storagetype: waijung_vdata_storage_callback('storagetype');
      mask Callback storagename: waijung_vdata_storage_callback('storagename');
      mask Callback initval: waijung_vdata_storage_callback('initval');
      mask Callback varname: waijung_vdata_storage_callback('varname');
      mask Callback initvalstring: waijung_vdata_storage_callback('initvalstring');
      mask TypeOptions webintegration: Disable | ReadOnly | Write/ Read | ReadOnly with KeyValuePair | Write/ Read with KeyValuePair
      mask Callback webintegration: waijung_vdata_storage_callback('webintegration');
      mask Callback weboutputformat: waijung_vdata_storage_callback('weboutputformat');
      mask TypeOptions laststoragetype: double | single | uint32 | int32 | uint16 | int16 | uint8 | int8 | string
      mask Callback sampletime: waijung_vdata_storage_callback('sampletime');
      mask Callback sampletimestr: waijung_vdata_storage_callback('sampletimestr');
      mask Callback blockid: waijung_vdata_storage_callback('blockid');
      mask Display: text(0.5, 0.5, 'Name: CircleR\nType: double','ver','middle','hor','center')
  flag_for_recorder_uart : S-Function  FunctionName=waijung_vdata_read  Parameters=storagename,varname,sampletime,sampletimestr,blockid,storagetype,storagetypestr  SFunctionDeploymentMode=off  EnableBusSupport=off  mask(waijung_vdata_read){storagename=flag, varname=VolatileDataStorage3_flag, sampletime=1e-2, sampletimestr=-1, blockid=flag_for_recorder_uart, storagetype=uint8, storagetypestr=uint8_t}
      mask prompts: storagename "Storage Name"; varname "Variable name"; sampletime "Sample time (sec)"; sampletimestr "Compiled sample time (sec) in string"; storagetype "Data type"; storagetypestr "Data type string"
      mask help: This block implements read data from a buffer.
      mask init:
      | waijung_vdata_read_callback('init');
      mask Help: web(fullfile(waijungdocroot,'Volatile_Data_Storage_Read.htm'))
      mask TypeOptions storagename: ab3 | ab1 | ab2 | ab4 | ab5 | ab6 | ab7 | ab8 | ab9 | ab10 | Ays | Ayc | Axs | A_Laser | LissaFreq | Axc | Laser | vcx | flag | CircleFlag | CircleFrequency | vcy | CircleR
      mask Callback storagename: waijung_vdata_read_callback('storagename');
      mask Callback varname: waijung_vdata_read_callback('varname');
      mask Callback sampletime: waijung_vdata_read_callback('sampletime');
      mask Callback sampletimestr: waijung_vdata_read_callback('sampletimestr');
      mask Callback blockid: waijung_vdata_read_callback('blockid');
      mask Callback storagetype: waijung_vdata_read_callback('storagetype');
      mask Display: text(0.05, 0.5, 'Buffer: flag','ver','middle','hor','left');port_label('output',1,'D1(uint8)')
  ignore_bad_data : Subsystem
  ignore_bad_data1 : Subsystem
  record_and_send_via_UART : Subsystem
  recording_clock : DiscretePulseGenerator  SampleTime=1e-2
  send_2_uart_clock : DiscretePulseGenerator  SampleTime=1e-2
  set_UART_VCflag : Subsystem
  wiggler : Subsystem
  wires:
  flag_for_recorder_uart/1 -> record_and_send_via_UART/5(flag_input)
  recording_clock/1 -> record_and_send_via_UART/6(record)
  send_2_uart_clock/1 -> record_and_send_via_UART/7(send)
  ignore_bad_data/1(Out1) -> Median Filter/1
  ignore_bad_data1/1(Out1) -> Median Filter1/1
  Median Filter/1 -> Index Vector/2
  Median Filter1/1 -> Index Vector1/2
  PWM chX/3 -> Sum/1
  Sum/1 -> ignore_bad_data/1(ADXL_X)
  Constant/1 -> Sum/2
  PWM chY/3 -> Sum1/1
  Sum1/1 -> ignore_bad_data1/1(ADXL_X)
  Constant1/1 -> Sum1/2
  [vc1] -> record_and_send_via_UART/3(In3)
  [vc2] -> record_and_send_via_UART/4(vc2)
  Index Vector/1 -> [adxl1]
  Index Vector1/1 -> [adxl2]
  [adxl1] -> record_and_send_via_UART/1(In1)
  [adxl2] -> record_and_send_via_UART/2(In2)
  Data Type Conversion/1 -> [vc2]
  Data Type Conversion1/1 -> [vc1]
  Volatile Data Storage Read2/1 -> Multiport Switch/1
  Multiport Switch/1 -> Demux/1
  Demux/1 -> Data Type Conversion1/1, wiggler/1(Motor2)
  Demux/2 -> Data Type Conversion/1, wiggler/2(Motor1)
  Calibration Vcx/1 -> Mux1/1
  Calibration Vcy/1 -> Mux1/2
  Mux1/1 -> Multiport Switch/2
  Circle/1(Circle Coordinates) -> Multiport Switch/3
  Lissajous/1(Lissajous Coordinates) -> Multiport Switch/4
